simulink model "GRPsimDragModel"  (R2024b)
settings: Solver=VariableStepAuto  StartTime=0.0  StopTime=10.0  RelTol=1e-3
libraries: shared6dof x1, aerolibasang x1, simulink x1, vrlib x1
settings Model: Creator=aniketray  LastModifiedBy=aniketray

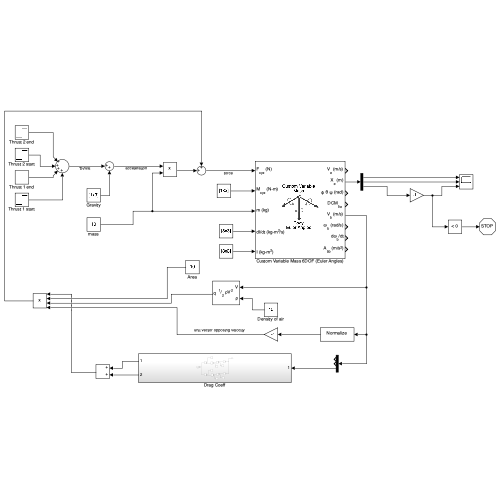
[thumbnail: Simulink's stored preview of the top-level diagram]
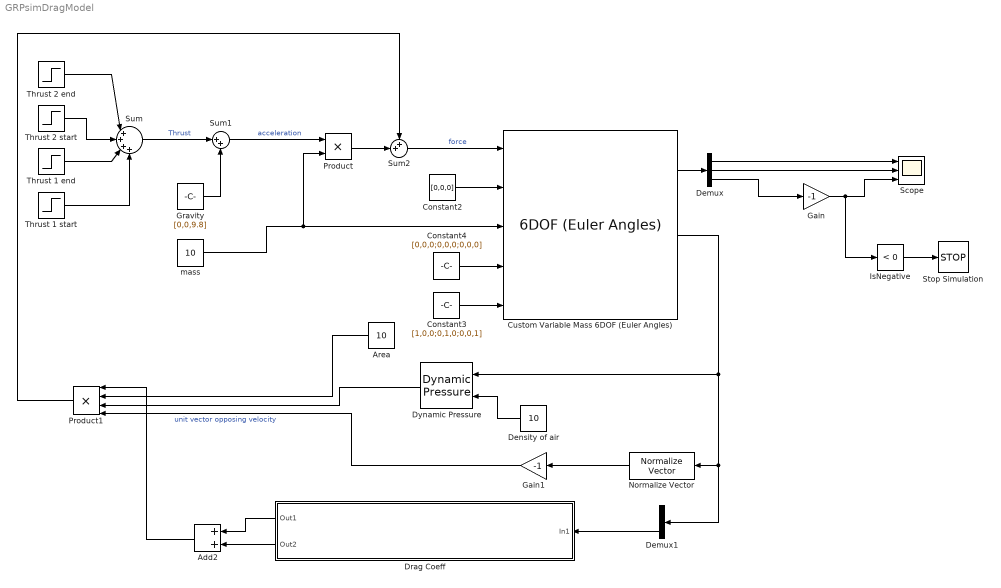
== system GRPsimDragModel ==
  Add2 : Sum
  Area : Constant  Value=10
  Constant2 : Constant  Value=[0,0,0]
  Constant3 : Constant  Value=[1,0,0;0,1,0;0,0,1]
  Constant4 : Constant  Value=[0,0,0;0,0,0;0,0,0]
  Custom Variable Mass 6DOF (Euler Angles) : shared6dof/6DOF (Euler Angles)  units=Metric (MKS)  mtype=Custom Variable  rep=Euler Angles  xme_0=[0 0 0]  Vm_0=[0 0 0]  eul_0=[0 0 0]  pm_0=[0 0 0]  mass_0=1.0  mass_e=0.5  mass_f=2.0  inertia=eye(3)  inertia_e=eye(3)  inertia_f=2*eye(3)  k_quat=1.0  vre_flag=off  abi_flag=off  aMode=0  xme_statename=''  Vm_statename=''  eul_statename=''  quat_statename=''  pm_statename=''  mass_statename=''
      settings: LibrarySourceBlock=aerolib6dof2/Custom Variable Mass 6DOF (Euler Angles)
  Demux : Demux  Outputs=3
  Demux1 : Demux  Outputs=3
  Density of air : Constant  Value=10
  Drag Coeff : Subsystem
  Dynamic Pressure : aerolibasang/Dynamic Pressure
  Gain : Gain  Gain=-1
  Gain1 : Gain  Gain=-1
  Gravity : Constant  Value=[0,0,9.8]
  IsNegative : simulink/Logic and Bit Operations/Compare To Zero  relop=<  OutDataTypeStr=boolean
      settings: LibrarySourceBlock=|
      | simulink/Quick Insert/Logic and Bit
      | Operations/IsNegative
  Normalize Vector : vrlib/Utilities/Normalize Vector  maxzero=0
  Product : Product
  Product1 : Product  Inputs=4
  Scope : Scope  NumInputPorts=3
  Stop Simulation : Stop
  Sum : Sum  Inputs=|++++
  Sum1 : Sum  Inputs=|++
  Sum2 : Sum  Inputs=++|
  Thrust 1 end : Step  Time=3  After=[0,0,15]  SampleTime=0.001
  Thrust 1 start : Step  Time=0  After=[0,0,-15]  SampleTime=0.001
  Thrust 2 end : Step  Time=9.1504293846  After=[0,0,15]  SampleTime=0.001
  Thrust 2 start : Step  Time=6.1504293846  After=[0,0,-15]  SampleTime=0.001
  mass : Constant  Value=10
  wires:
  Demux/3 -> Gain/1
  Gravity/1 -> Sum1/2
  mass/1 -> Custom Variable Mass 6DOF (Euler Angles)/3, Product/2
  Sum/1 -> Sum1/1  "Thrust"
  Constant3/1 -> Custom Variable Mass 6DOF (Euler Angles)/5
  Demux/2 -> Scope/2
  Thrust 2 end/1 -> Sum/1
  IsNegative/1 -> Stop Simulation/1
  Custom Variable Mass 6DOF (Euler Angles)/2 -> Demux/1
  Demux/1 -> Scope/1
  Thrust 1 end/1 -> Sum/3
  Constant2/1 -> Custom Variable Mass 6DOF (Euler Angles)/2
  Constant4/1 -> Custom Variable Mass 6DOF (Euler Angles)/4
  Sum1/1 -> Product/1  "acceleration"
  Thrust 2 start/1 -> Sum/2
  Thrust 1 start/1 -> Sum/4
  Gain/1 -> IsNegative/1, Scope/3
  Dynamic Pressure/1 -> Product1/3
  Area/1 -> Product1/2
  Custom Variable Mass 6DOF (Euler Angles)/5 -> Demux1/1, Normalize Vector/1, Dynamic Pressure/1
  Density of air/1 -> Dynamic Pressure/2
  Product/1 -> Sum2/2
  Normalize Vector/1 -> Gain1/1
  Gain1/1 -> Product1/4  "unit vector opposing velocity"
  Sum2/1 -> Custom Variable Mass 6DOF (Euler Angles)/1  "force"
  Add2/1 -> Product1/1
  Demux1/3 -> Drag Coeff/1(In1)
  Drag Coeff/1(Out1) -> Add2/1
  Drag Coeff/2(Out2) -> Add2/2
  Product1/1 -> Sum2/1

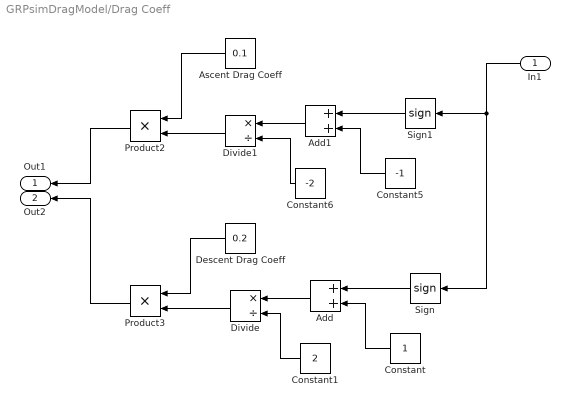
== system GRPsimDragModel/Drag Coeff ==
  In1 : Inport
  Add : Sum
  Add1 : Sum
  Ascent Drag Coeff : Constant  Value=0.1
  Constant : Constant
  Constant1 : Constant  Value=2
  Constant5 : Constant  Value=-1
  Constant6 : Constant  Value=-2
  Descent Drag Coeff : Constant  Value=0.2
  Divide : Product  Inputs=*/
  Divide1 : Product  Inputs=*/
  Product2 : Product
  Product3 : Product
  Sign : Signum
  Sign1 : Signum
  Out1 : Outport
  Out2 : Outport  Port=2
  wires:
  Product2/1 -> Out1/1
  Descent Drag Coeff/1 -> Product3/1
  Divide1/1 -> Product2/2
  Constant/1 -> Add/2
  Constant1/1 -> Divide/2
  Add1/1 -> Divide1/1
  Divide/1 -> Product3/2
  Add/1 -> Divide/1
  Ascent Drag Coeff/1 -> Product2/1
  Sign1/1 -> Add1/1
  Constant5/1 -> Add1/2
  Product3/1 -> Out2/1
  Constant6/1 -> Divide1/2
  In1/1 -> Sign1/1, Sign/1
  Sign/1 -> Add/1
